simulink subsystem "FIRReferenceGenerator"  (R2025b)
settings: Solver=VariableStepAuto  StartTime=0.0  StopTime=10.0  RelTol=1e-3
undefined symbols (not defined in the file or in its folder): A_bar, Ts
settings Model: Creator=leeta  LastModifiedBy=leeta

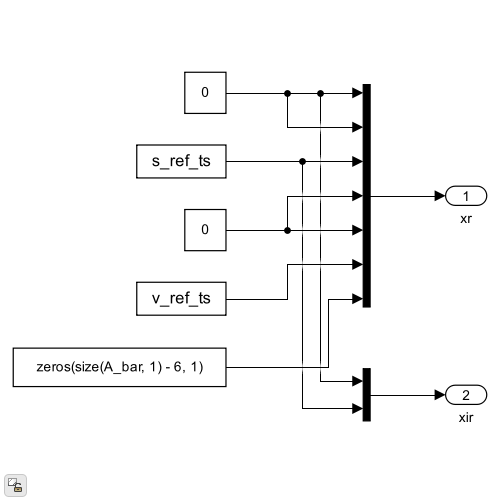
[thumbnail: Simulink's stored preview of the top-level diagram]
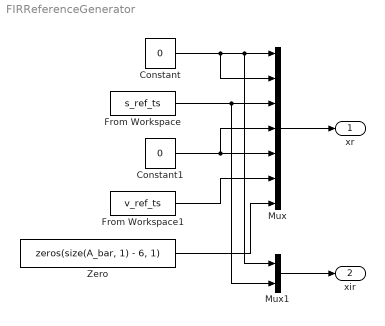
== system FIRReferenceGenerator ==
  Constant : Constant  Value=0
  Constant1 : Constant  Value=0
  From Workspace : FromWorkspace  VariableName=s_ref_ts  SampleTime=Ts
  From Workspace1 : FromWorkspace  VariableName=v_ref_ts  SampleTime=Ts
  Mux : Mux  Inputs=7
  Mux1 : Mux  Inputs=2
  Zero : Constant  Value=zeros(size(A_bar, 1) - 6, 1)
  xr : Outport
  xir : Outport  Port=2
  wires:
  Mux/1 -> xr/1
  Constant/1 -> Mux/1, Mux1/1, Mux/2
  From Workspace/1 -> Mux1/2, Mux/3
  Constant1/1 -> Mux/4, Mux/5
  From Workspace1/1 -> Mux/6
  Zero/1 -> Mux/7
  Mux1/1 -> xir/1
